simulink model "ku_method_1"  (R2023b)
settings: Solver=VariableStepAuto  StartTime=0.0  StopTime=10.0  RelTol=1e-3
settings Model: Creator=hmvke  LastModifiedBy=hmvke

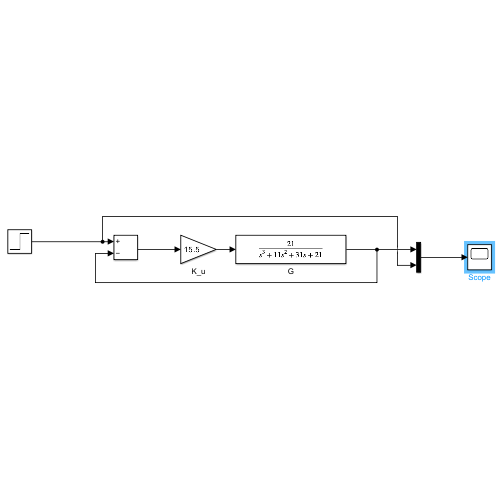
[thumbnail: Simulink's stored preview of the top-level diagram]
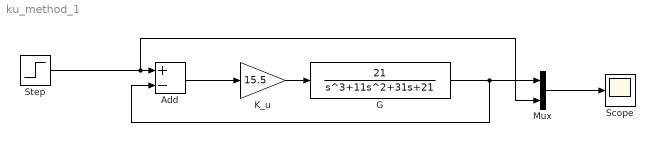
== system ku_method_1 ==
  Add : Sum  Inputs=+-
  G : TransferFcn  Numerator=[21]  Denominator=[1 11 31 21]
  K_u : Gain  Gain=15.5
  Mux : Mux  Inputs=2
  Scope : Scope
  Step : Step  SampleTime=0
  wires:
  Step/1 -> Mux/2, Add/1
  Add/1 -> K_u/1
  K_u/1 -> G/1
  G/1 -> Mux/1, Add/2
  Mux/1 -> Scope/1
